simulink model "combine"  (R2017b)
settings: Solver=VariableStepAuto  StartTime=0.0  StopTime=10.0  FixedStep=0.1  RelTol=1e-3  EnableMultiTasking=on
values from neighbouring files (symbols this model uses):
  A = [0 1 0 0 ... (first row only)    [final.m]    (also in parameter.m)
  B = [0; B_2; 0; B_4]    [final.m]    (also in parameter.m)
  C = eye(4)    [final.m]    (also in parameter.m)
  D = zeros(4, 1)    [final.m]    (also in parameter.m)
  K = place(A, B, pole_desired)    [final.m]
  L = transpose(L)    [final.m]    (also in parameter.m = 0.11)
  xhatini = xini    [final.m]
  xini = [0; 0; 0; 0]    [final.m]
settings Model: Creator=hrlin  LastModifiedBy=Administrator
settings DataIOCC: LimitDataPoints=on  SaveFormat=Array  SignalLoggingSaveFormat=ModelDataLogs
settings OptimizationCC: InitFltsAndDblsToZero=on  LifeSpan=inf
settings DebuggingCC: SaveWithParameterizedLinksMsg=none  UnderspecifiedInitializationDetection=Classic  MergeDetectMultiDrivingBlocksExec=none  SignalResolutionControl=TryResolveAllWithWarning  MultiTaskDSMMsg=warning  MultiTaskCondExecSysMsg=none  FcnCallInpInsideContextMsg=warning  SFUnexpectedBacktrackingDiag=warning  SFNoUnconditionalDefaultTransitionDiag=warning  SFExecutionAtInitializationDiag=none
settings HardwareCC: ProdBitPerPointer=32  ProdBitPerSizeT=32  ProdBitPerPtrDiffT=32  ProdLargestAtomicFloat=None  ProdIntDivRoundTo=Undefined  ProdEndianess=Unspecified  ProdWordSize=32  ProdHWDeviceType=32-bit Generic
settings ModelReferenceCC: PropagateSignalLabelsOutOfModel=off
settings CodeAppCC: StateflowObjectComments=on
settings GRTTargetCC: TargetFcnLib=ansi_tfl_tmw.mat  TargetLangStandard=C89/C90 (ANSI)  GeneratePreprocessorConditionals=Disable all  CombineOutputUpdateFcns=off  GRTInterface=on
settings ConfigComp: CovMetricSettings=dw  CovHtmlReporting=on  CovSaveCumulativeToWorkspaceVar=on  CovSaveSingleToWorkspaceVar=on  CovExternalEMLEnable=off

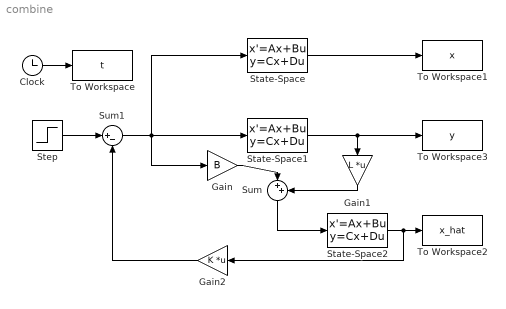
== system combine ==
  Clock : Clock
  Gain : Gain  Gain=B
  Gain1 : Gain  Gain=L  Multiplication=Matrix(K*u)
  Gain2 : Gain  Gain=K  Multiplication=Matrix(K*u)
  State-Space : StateSpace  A=A  B=B  C=eye(size(A))  D=zeros(size(C,1),size(B,2))  InitialCondition=xini
  State-Space1 : StateSpace  A=A  B=B  C=C  D=D  InitialCondition=xini
  State-Space2 : StateSpace  A=A-L*C  B=eye(4)  C=eye(4)  D=zeros(4,4)  InitialCondition=xhatini
  Step : Step  SampleTime=0
  Sum : Sum  Inputs=|++
  Sum1 : Sum  Inputs=|+-
  To Workspace : ToWorkspace  VariableName=t  SampleTime=-1
  To Workspace1 : ToWorkspace  VariableName=x  SampleTime=-1
  To Workspace2 : ToWorkspace  VariableName=x_hat  SampleTime=-1
  To Workspace3 : ToWorkspace  VariableName=y  SampleTime=-1
  wires:
  Clock/1 -> To Workspace/1
  State-Space/1 -> To Workspace1/1
  State-Space1/1 -> Gain1/1, To Workspace3/1
  Gain/1 -> Sum/1
  Gain1/1 -> Sum/2
  Sum/1 -> State-Space2/1
  State-Space2/1 -> Gain2/1, To Workspace2/1
  Step/1 -> Sum1/1
  Sum1/1 -> Gain/1, State-Space/1, State-Space1/1
  Gain2/1 -> Sum1/2
